simulink model "MultirotorSimPx4v1_8ContMatrix"  (R2018b)
settings: Solver=ode45  StartTime=0.0  StopTime=Simulation.T_END  MaxStep=Simulation.TS_MAX  RelTol=1e-3  EnableMultiTasking=on
PreLoadFcn:
  | % InitializeParameters;
undefined symbols (not defined in the file): Ctrl, Initial, Kpid, Uav, Wind
libraries: QuaternionLibrary x13, simulink x5, simulink_extras x4
(part 2 of 2)

== system MultirotorSimPx4v1_8ContMatrix/Hinf Controller/2D Rotation Matrix ==
  psi : Inport
  Cos : Trigonometry  Operator=cos
  Cos1 : Trigonometry
  Cos2 : Trigonometry
  Cos3 : Trigonometry  Operator=cos
  Gain : Gain  Gain=-1
  Matrix Concatenate : Concatenate  Mode=Multidimensional array  ConcatenateDimension=2
  Mux : Mux  Inputs=2
  Mux1 : Mux  Inputs=2
  R : Outport
  wires:
  Cos3/1 -> Mux1/2
  Cos2/1 -> Mux1/1
  Mux/1 -> Matrix Concatenate/1
  Cos1/1 -> Gain/1
  Cos/1 -> Mux/1
  Gain/1 -> Mux/2
  Mux1/1 -> Matrix Concatenate/2
  Matrix Concatenate/1 -> R/1
  psi/1 -> Cos/1, Cos1/1, Cos2/1, Cos3/1

== system MultirotorSimPx4v1_8ContMatrix/Pos Control/Filtered Derivative ==
  xiDot : Inport  Unit=m/s
  D filter x : TransferFcn  Denominator=[1/(PID_FC*2*pi) 1]  ContinuousStateAttributes='velPID_D_x'
  D filter y : TransferFcn  Denominator=[1/(PID_FC*2*pi) 1]  ContinuousStateAttributes='velPID_D_y'
  D filter z : TransferFcn  Denominator=[1/(PID_FC*2*pi) 1]  ContinuousStateAttributes='velPID_D_z'
  Demux : Demux  Outputs=3
  Mux2 : Mux  Inputs=3
  xiDDotF : Outport  Unit=m/s^2
  wires:
  D filter x/1 -> Mux2/1
  Demux/2 -> D filter y/1
  D filter y/1 -> Mux2/2
  xiDot/1 -> Demux/1
  D filter z/1 -> Mux2/3
  Demux/1 -> D filter x/1
  Demux/3 -> D filter z/1
  Mux2/1 -> xiDDotF/1

== system MultirotorSimPx4v1_8ContMatrix/Pos Control/Filtered Derivative1 ==
  xiDot : Inport  Unit=m/s
  D filter x : TransferFcn  Numerator=[1 0]  Denominator=[1/(PID_FC*2*pi) 1]  ContinuousStateAttributes='velPID_D_x'
  D filter y : TransferFcn  Numerator=[1 0]  Denominator=[1/(PID_FC*2*pi) 1]  ContinuousStateAttributes='velPID_D_y'
  D filter z : TransferFcn  Numerator=[1 0]  Denominator=[1/(PID_FC*2*pi) 1]  ContinuousStateAttributes='velPID_D_z'
  Demux : Demux  Outputs=3
  Mux2 : Mux  Inputs=3
  xiDDotF : Outport  Unit=m/s^2
  wires:
  Mux2/1 -> xiDDotF/1
  Demux/3 -> D filter z/1
  Demux/1 -> D filter x/1
  D filter z/1 -> Mux2/3
  xiDot/1 -> Demux/1
  D filter y/1 -> Mux2/2
  Demux/2 -> D filter y/1
  D filter x/1 -> Mux2/1

== system MultirotorSimPx4v1_8ContMatrix/Pos Control/x vel PID ==
  ref : Inport
  meas : Inport  Port=2
  Add : Sum  Inputs=++-
  D : Gain  Gain=PID_D
  D filter : TransferFcn  Numerator=[1 0]  Denominator=[1/(PID_FC*2*pi) 1]  ContinuousStateAttributes=PID_D_STATENAME
  I : Gain  Gain=PID_I
  Integrator1 : Integrator  UpperSaturationLimit=0.3  LowerSaturationLimit=-0.3  ContinuousStateAttributes=PID_I_STATENAME
  P : Gain  Gain=PID_P
  Sum : Sum  Inputs=|+-
  Out : Outport
  wires:
  Add/1 -> Out/1
  P/1 -> Add/1
  Integrator1/1 -> Add/2
  D filter/1 -> D/1
  Sum/1 -> I/1, P/1
  D/1 -> Add/3
  I/1 -> Integrator1/1
  ref/1 -> Sum/1
  meas/1 -> D filter/1, Sum/2

== system MultirotorSimPx4v1_8ContMatrix/Pos Control/y vel PID ==
  ref : Inport
  meas : Inport  Port=2
  Add : Sum  Inputs=++-
  D : Gain  Gain=PID_D
  D filter : TransferFcn  Numerator=[1 0]  Denominator=[1/(PID_FC*2*pi) 1]  ContinuousStateAttributes=PID_D_STATENAME
  I : Gain  Gain=PID_I
  Integrator1 : Integrator  UpperSaturationLimit=0.3  LowerSaturationLimit=-0.3  ContinuousStateAttributes=PID_I_STATENAME
  P : Gain  Gain=PID_P
  Sum : Sum  Inputs=|+-
  Out : Outport
  wires:
  meas/1 -> Sum/2, D filter/1
  ref/1 -> Sum/1
  I/1 -> Integrator1/1
  D/1 -> Add/3
  Sum/1 -> P/1, I/1
  D filter/1 -> D/1
  Integrator1/1 -> Add/2
  P/1 -> Add/1
  Add/1 -> Out/1

== system MultirotorSimPx4v1_8ContMatrix/Pos Control/z vel PID ==
  ref : Inport
  meas : Inport  Port=2
  Add : Sum  Inputs=++-
  D : Gain  Gain=PID_D
  D filter : TransferFcn  Numerator=[1 0]  Denominator=[1/(PID_FC*2*pi) 1]  ContinuousStateAttributes=PID_D_STATENAME
  I : Gain  Gain=PID_I
  Integrator1 : Integrator  UpperSaturationLimit=0.3  LowerSaturationLimit=-0.3  ContinuousStateAttributes=PID_I_STATENAME
  P : Gain  Gain=PID_P
  Sum : Sum  Inputs=|+-
  Out : Outport
  wires:
  Add/1 -> Out/1
  P/1 -> Add/1
  Integrator1/1 -> Add/2
  D filter/1 -> D/1
  Sum/1 -> I/1, P/1
  D/1 -> Add/3
  I/1 -> Integrator1/1
  ref/1 -> Sum/1
  meas/1 -> D filter/1, Sum/2

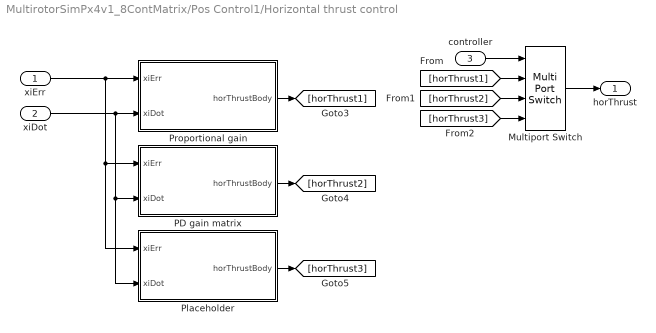
== system MultirotorSimPx4v1_8ContMatrix/Pos Control1/Horizontal thrust control ==
  "xiErr " : Inport
  "xiDot " : Inport  Port=2
  controller : Inport  Port=3
  Multiport Switch : MultiPortSwitch
  PD gain matrix : Subsystem  VariantControl=HorThrustWorldFrame
  Placeholder : Subsystem  VariantControl=HorThrustWorldFrame
  Proportional gain : Subsystem  VariantControl=HorThrustWorldFrame
  " horThrust" : Outport
  wires:
  "xiErr "/1 -> PD gain matrix/1("xiErr "), Placeholder/1("xiErr "), Proportional gain/1("xiErr ")
  "xiDot "/1 -> Proportional gain/2("xiDot "), PD gain matrix/2(xiDot), Placeholder/2(xiDot)
  Multiport Switch/1 -> " horThrust"/1
  controller/1 -> Multiport Switch/1
  Proportional gain/1(" horThrustBody") -> [horThrust1]
  PD gain matrix/1(" horThrustBody") -> [horThrust2]
  Placeholder/1(" horThrustBody") -> [horThrust3]
  [horThrust1] -> Multiport Switch/2
  [horThrust2] -> Multiport Switch/3
  [horThrust3] -> Multiport Switch/4

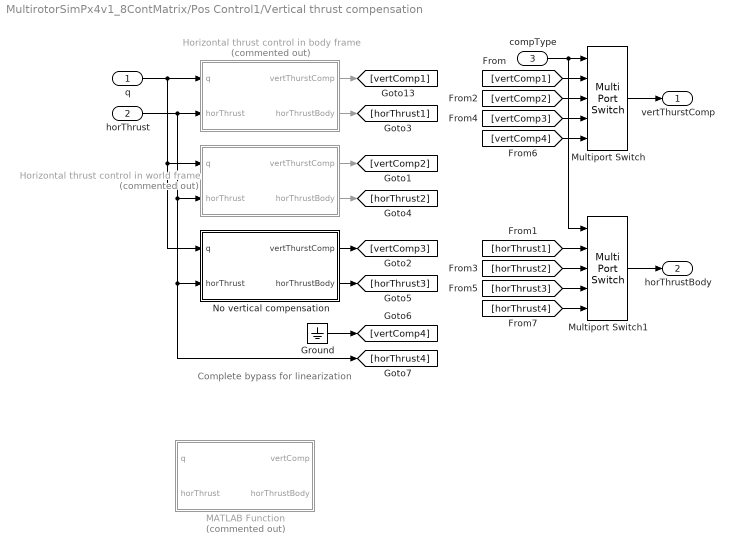
== system MultirotorSimPx4v1_8ContMatrix/Pos Control1/Vertical thrust compensation ==
  note: Complete bypass for linearization
  "q " : Inport
  "horThrust " : Inport  Port=2
  compType : Inport  Port=3
  Ground : Ground
  Horizontal thrust control in body frame : Subsystem  Commented=on  VariantControl=HorThrustBodyFrame
  Horizontal thrust control in world frame : Subsystem  Commented=on  VariantControl=HorThrustWorldFrame
  MATLAB Function : MATLAB Function  Commented=on  TreatAsAtomicUnit=on
  Multiport Switch : MultiPortSwitch  Inputs=4
  Multiport Switch1 : MultiPortSwitch  Inputs=4
  No vertical compensation : Subsystem  VariantControl=HorThrustNoVertComp
  " vertThurstComp" : Outport
  " horThrustBody" : Outport  Port=2
  wires:
  Ground/1 -> [vertComp4]
  [horThrust4] -> Multiport Switch1/5
  [vertComp4] -> Multiport Switch/5
  [horThrust1] -> Multiport Switch1/2
  [horThrust2] -> Multiport Switch1/3
  [horThrust3] -> Multiport Switch1/4
  [vertComp3] -> Multiport Switch/4
  [vertComp2] -> Multiport Switch/3
  [vertComp1] -> Multiport Switch/2
  No vertical compensation/2(" horThrustBody") -> [horThrust3]
  Horizontal thrust control in world frame/2(" horThrustBody") -> [horThrust2]
  Horizontal thrust control in body frame/2(horThrustBody) -> [horThrust1]
  No vertical compensation/1(" vertThurstComp") -> [vertComp3]
  Horizontal thrust control in world frame/1(" vertThurstComp") -> [vertComp2]
  Horizontal thrust control in body frame/1(vertThurstComp) -> [vertComp1]
  compType/1 -> Multiport Switch/1, Multiport Switch1/1
  Multiport Switch1/1 -> " horThrustBody"/1
  Multiport Switch/1 -> " vertThurstComp"/1
  "horThrust "/1 -> Horizontal thrust control in body frame/2(horThrust), Horizontal thrust control in world frame/2("horThrust "), No vertical compensation/2("horThrust "), [horThrust4]
  "q "/1 -> Horizontal thrust control in body frame/1(q), Horizontal thrust control in world frame/1("q "), No vertical compensation/1("q ")

== system MultirotorSimPx4v1_8ContMatrix/Pos Control1/Horizontal thrust control/PD gain matrix ==
  "xiErr " : Inport
  xiDot : Inport  Port=2
  HT_xDotYDot : Gain  Gain=-0.001
  HT_xy : Gain  Gain=0.01
  Selector : Selector  InputPortWidth=3  IndexOptions=Index vector (dialog)  Indices=[1 2]  OutputSizes=1
  Selector1 : Selector  InputPortWidth=3  IndexOptions=Index vector (dialog)  Indices=[1 2]  OutputSizes=1
  Sum : Sum  Inputs=|++
  " horThrustBody" : Outport
  wires:
  Sum/1 -> " horThrustBody"/1
  HT_xDotYDot/1 -> Sum/2
  HT_xy/1 -> Sum/1
  Selector1/1 -> HT_xDotYDot/1
  Selector/1 -> HT_xy/1
  xiDot/1 -> Selector1/1
  "xiErr "/1 -> Selector/1

== system MultirotorSimPx4v1_8ContMatrix/Pos Control1/Horizontal thrust control/Placeholder ==
  "xiErr " : Inport
  xiDot : Inport  Port=2
  C : simulink/Continuous/PID Controller  Controller=PD  Form=Parallel  TimeDomain=Continuous-time  SampleTime=-1  IntegratorMethod=Forward Euler  FilterMethod=Forward Euler  ControllerParametersSource=internal  P=3.97886854580772  I=1  D=0.19015657256146  UseFilter=on  N=18.1835914295571  TunerSelectOption=Transfer Function Based (PID Tuner App)  InitialConditionSource=internal  InitialConditionForIntegrator=0  InitialConditionForFilter=0  DifferentiatorICPrevScaledInput=0  ExternalReset=none  TrackingMode=off  Kt=1  LimitOutput=off  UpperSaturationLimit=inf  LowerSaturationLimit=-inf  LinearizeAsGain=on  AntiWindupMode=none  Kb=1  POutMin=[]  POutMax=[]  IOutMin=[]  IOutMax=[]  DOutMin=[]  DOutMax=[]  NOutMin=[]  NOutMax=[]  SumOutMin=[]  SumOutMax=[]  SaturationOutMin=[]  SaturationOutMax=[]  PParamMin=[]  PParamMax=[]  IParamMin=[]  IParamMax=[]  DParamMin=[]  DParamMax=[]  NParamMin=[]  NParamMax=[]  KbParamMin=[]  KbParamMax=[]  KtParamMin=[]  KtParamMax=[]  KbOutMin=[]  KbOutMax=[]  KtOutMin=[]  KtOutMax=[]  IntegratorOutMin=[]  IntegratorOutMax=[]  FilterOutMin=[]  FilterOutMax=[]  SumI1OutMin=[]  SumI1OutMax=[]  SumI2OutMin=[]  SumI2OutMax=[]  SumI3OutMin=[]  SumI3OutMax=[]  SumI4OutMin=[]  SumI4OutMax=[]  SumDOutMin=[]  SumDOutMax=[]  DifferentiatorOutMin=[]  DifferentiatorOutMax=[]  FilterDiffOutCoefMin=[]  FilterDiffOutCoefMax=[]  ReciprocalOutMin=[]  ReciprocalOutMax=[]  SumDenOutMin=[]  SumDenOutMax=[]  SumNumOutMin=[]  SumNumOutMax=[]  DivideOutMin=[]  DivideOutMax=[]  IntegratorContinuousStateAttributes=''  IntegratorStateMustResolveToSignalObject=off  IntegratorRTWStateStorageClass=Auto  FilterContinuousStateAttributes=''  FilterStateMustResolveToSignalObject=off  FilterRTWStateStorageClass=Auto  ParallelPVariant=InternalParameters  IdealPVariant=Disabled  IVariant=Disabled  DVariant=InternalParameters  IntegratorVariant=Disabled  SatVariant=Disabled  AWVariant=Disabled  PCopyVariant=Disabled  TRVariant=Disabled  FdbkBlocksVariant=Forward  IdealPFdbkVariant=Disabled  SatFdbkVariant=Disabled  DerivativeFilterVariant=ContFilter  NVariant=InternalParameters  NCopyVariant=Disabled  FilterICVariant=InternalICsFilter  IntegratorICVariant=Disabled  ExternalResetVariant=Disabled  TRSumVariant=Passthrough  SumFdbkVariant=Disabled  SumVariant=Sum_PD
  C1 : simulink/Continuous/PID Controller  Controller=PD  Form=Parallel  TimeDomain=Continuous-time  SampleTime=-1  IntegratorMethod=Forward Euler  FilterMethod=Forward Euler  ControllerParametersSource=internal  P=3.97886854580772  I=1  D=0.19015657256146  UseFilter=on  N=18.1835914295571  TunerSelectOption=Transfer Function Based (PID Tuner App)  InitialConditionSource=internal  InitialConditionForIntegrator=0  InitialConditionForFilter=0  DifferentiatorICPrevScaledInput=0  ExternalReset=none  TrackingMode=off  Kt=1  LimitOutput=off  UpperSaturationLimit=inf  LowerSaturationLimit=-inf  LinearizeAsGain=on  AntiWindupMode=none  Kb=1  POutMin=[]  POutMax=[]  IOutMin=[]  IOutMax=[]  DOutMin=[]  DOutMax=[]  NOutMin=[]  NOutMax=[]  SumOutMin=[]  SumOutMax=[]  SaturationOutMin=[]  SaturationOutMax=[]  PParamMin=[]  PParamMax=[]  IParamMin=[]  IParamMax=[]  DParamMin=[]  DParamMax=[]  NParamMin=[]  NParamMax=[]  KbParamMin=[]  KbParamMax=[]  KtParamMin=[]  KtParamMax=[]  KbOutMin=[]  KbOutMax=[]  KtOutMin=[]  KtOutMax=[]  IntegratorOutMin=[]  IntegratorOutMax=[]  FilterOutMin=[]  FilterOutMax=[]  SumI1OutMin=[]  SumI1OutMax=[]  SumI2OutMin=[]  SumI2OutMax=[]  SumI3OutMin=[]  SumI3OutMax=[]  SumI4OutMin=[]  SumI4OutMax=[]  SumDOutMin=[]  SumDOutMax=[]  DifferentiatorOutMin=[]  DifferentiatorOutMax=[]  FilterDiffOutCoefMin=[]  FilterDiffOutCoefMax=[]  ReciprocalOutMin=[]  ReciprocalOutMax=[]  SumDenOutMin=[]  SumDenOutMax=[]  SumNumOutMin=[]  SumNumOutMax=[]  DivideOutMin=[]  DivideOutMax=[]  IntegratorContinuousStateAttributes=''  IntegratorStateMustResolveToSignalObject=off  IntegratorRTWStateStorageClass=Auto  FilterContinuousStateAttributes=''  FilterStateMustResolveToSignalObject=off  FilterRTWStateStorageClass=Auto  ParallelPVariant=InternalParameters  IdealPVariant=Disabled  IVariant=Disabled  DVariant=InternalParameters  IntegratorVariant=Disabled  SatVariant=Disabled  AWVariant=Disabled  PCopyVariant=Disabled  TRVariant=Disabled  FdbkBlocksVariant=Forward  IdealPFdbkVariant=Disabled  SatFdbkVariant=Disabled  DerivativeFilterVariant=ContFilter  NVariant=InternalParameters  NCopyVariant=Disabled  FilterICVariant=InternalICsFilter  IntegratorICVariant=Disabled  ExternalResetVariant=Disabled  TRSumVariant=Passthrough  SumFdbkVariant=Disabled  SumVariant=Sum_PD
  Mux : Mux  Inputs=2
  Selector : Selector  InputPortWidth=3  IndexOptions=Index vector (dialog)  Indices=[1]  OutputSizes=1
  Selector1 : Selector  InputPortWidth=3  IndexOptions=Index vector (dialog)  Indices=[2]  OutputSizes=1
  Terminator1 : Terminator
  " horThrustBody" : Outport
  wires:
  C/1 -> Mux/1  "u"
  C1/1 -> Mux/2  "u"
  Selector/1 -> C/1
  Selector1/1 -> C1/1
  Mux/1 -> " horThrustBody"/1
  xiDot/1 -> Terminator1/1
  "xiErr "/1 -> Selector1/1, Selector/1

== system MultirotorSimPx4v1_8ContMatrix/Pos Control1/Horizontal thrust control/Proportional gain ==
  "xiErr " : Inport
  "xiDot " : Inport  Port=2
  Selector : Selector  InputPortWidth=3  IndexOptions=Index vector (dialog)  Indices=[1 2]  OutputSizes=1
  Terminator : Terminator
  hor_xy : Gain  Gain=Ctrl.HOR_GAIN
  " horThrustBody" : Outport
  wires:
  Selector/1 -> hor_xy/1
  "xiDot "/1 -> Terminator/1
  hor_xy/1 -> " horThrustBody"/1
  "xiErr "/1 -> Selector/1

== system MultirotorSimPx4v1_8ContMatrix/Pos Control1/Vertical thrust compensation/Horizontal thrust control in body frame ==
  q : Inport
  horThrust : Inport  Port=2
  2D Rotation Matrix : Subsystem
  Matrix Multiply : Product  Multiplication=Matrix(*)
  Quaternion to Euler Angles : QuaternionLibrary/Quaternion to Euler Angles
  Selector : Selector  InputPortWidth=3  IndexOptions=Index vector (dialog)  Indices=3  OutputSizes=1
  Subsystem : Subsystem
  vertThurstComp : Outport
  horThrustBody : Outport  Port=2
  wires:
  Matrix Multiply/1 -> horThrustBody/1
  2D Rotation Matrix/1(R) -> Matrix Multiply/1
  Selector/1 -> 2D Rotation Matrix/1(psi)
  Subsystem/1(thrustComp) -> vertThurstComp/1
  Quaternion to Euler Angles/1 -> Selector/1
  q/1 -> Subsystem/1(q), Quaternion to Euler Angles/1
  horThrust/1 -> Subsystem/2(horThrust), Matrix Multiply/2

== system MultirotorSimPx4v1_8ContMatrix/Pos Control1/Vertical thrust compensation/Horizontal thrust control in world frame ==
  "q " : Inport
  "horThrust " : Inport  Port=2
  Demux : Demux  Outputs=3
  Gain : Gain  Commented=through  Gain=-1
  Matrix Multiply1 : Product  Multiplication=Matrix(*)
  Mux : Mux  Inputs=2
  Mux1 : Mux  Inputs=2
  Quaternion to Rotation Matrix : QuaternionLibrary/Quaternion to Rotation Matrix
  Transpose : Math  Operator=transpose  SaturateOnIntegerOverflow=on
  z element : Constant  Value=0
  " vertThurstComp" : Outport
  " horThrustBody" : Outport  Port=2
  wires:
  Transpose/1 -> Matrix Multiply1/1
  Gain/1 -> " vertThurstComp"/1
  Demux/3 -> Gain/1
  Mux1/1 -> " horThrustBody"/1
  Demux/1 -> Mux1/1
  Demux/2 -> Mux1/2
  Matrix Multiply1/1 -> Demux/1  "horThurstBody"
  Quaternion to Rotation Matrix/1 -> Transpose/1
  "q "/1 -> Quaternion to Rotation Matrix/1
  "horThrust "/1 -> Mux/1
  z element/1 -> Mux/2
  Mux/1 -> Matrix Multiply1/2

== system MultirotorSimPx4v1_8ContMatrix/Pos Control1/Vertical thrust compensation/No vertical compensation ==
  "q " : Inport
  "horThrust " : Inport  Port=2
  2D Rotation Matrix : Subsystem
  Ground : Ground
  Matrix Multiply : Product  Multiplication=Matrix(*)
  Quaternion to Euler Angles : QuaternionLibrary/Quaternion to Euler Angles
  Scope : Scope
  Selector : Selector  InputPortWidth=3  IndexOptions=Index vector (dialog)  Indices=3  OutputSizes=1
  " vertThurstComp" : Outport
  " horThrustBody" : Outport  Port=2
  wires:
  "horThrust "/1 -> Matrix Multiply/2
  Quaternion to Euler Angles/1 -> Selector/1
  Selector/1 -> 2D Rotation Matrix/1(psi), Scope/1
  "q "/1 -> Quaternion to Euler Angles/1
  2D Rotation Matrix/1(R) -> Matrix Multiply/1
  Ground/1 -> " vertThurstComp"/1
  Matrix Multiply/1 -> " horThrustBody"/1

== system MultirotorSimPx4v1_8ContMatrix/Pos Control1/Vertical thrust compensation/Horizontal thrust control in body frame/2D Rotation Matrix ==
  psi : Inport
  Cos : Trigonometry  Operator=cos
  Cos1 : Trigonometry
  Cos2 : Trigonometry
  Cos3 : Trigonometry  Operator=cos
  Display : Display
  Gain : Gain  Gain=-1
  Matrix Concatenate : Concatenate  Mode=Multidimensional array  ConcatenateDimension=2
  Mux : Mux  Inputs=2
  Mux1 : Mux  Inputs=2
  R : Outport
  wires:
  psi/1 -> Cos3/1, Cos2/1, Cos1/1, Cos/1
  Matrix Concatenate/1 -> R/1, Display/1
  Mux1/1 -> Matrix Concatenate/2
  Gain/1 -> Mux/2
  Cos/1 -> Mux/1
  Cos1/1 -> Gain/1
  Mux/1 -> Matrix Concatenate/1
  Cos2/1 -> Mux1/1
  Cos3/1 -> Mux1/2

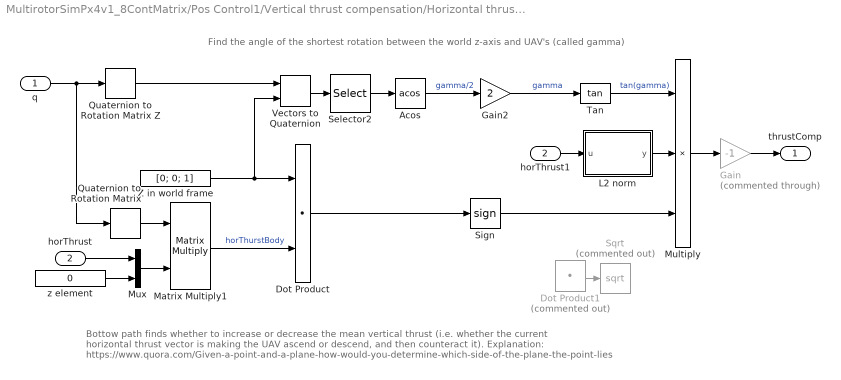
== system MultirotorSimPx4v1_8ContMatrix/Pos Control1/Vertical thrust compensation/Horizontal thrust control in body frame/Subsystem ==
  note: Bottow path finds whether to increase or decrease the mean vertical thrust (i.e. whether the current horizontal thrust vector is
      | making the UAV ascend or descend, and then counteract it).
      | Explanation: https://www.quora.com/Given-a-point-and-a-plane-how-would-you-determine-which-side-of-the-plane-the-point-lies
  note: Find the angle of the shortest rotation between the world z-axis and UAV's (called gamma)
  q : Inport
  horThrust : Inport  Port=2
  Acos : Trigonometry  Operator=acos
  Dot Product : DotProduct  InputSameDT=on  OutDataTypeStr=Inherit: Inherit via internal rule
  Dot Product1 : DotProduct  Commented=on  InputSameDT=on  OutDataTypeStr=Inherit: Inherit via internal rule
  Gain : Gain  Commented=through  Gain=-1
  Gain2 : Gain  Gain=2
  L2 norm : MATLAB Function  TreatAsAtomicUnit=on
  Matrix Multiply1 : Product  Multiplication=Matrix(*)
  Multiply : Product  Inputs=***
  Mux : Mux  Inputs=2
  Quaternion to Rotation Matrix : QuaternionLibrary/Quaternion to Rotation Matrix
  Quaternion to Rotation Matrix Z : QuaternionLibrary/Quaternion to Rotation Matrix Z
  Selector2 : Selector  InputPortWidth=4  IndexOptions=Index vector (dialog)  Indices=1  OutputSizes=1
  Sign : Signum
  Sqrt : Sqrt  Commented=on  SaturateOnIntegerOverflow=on
  Tan : Trigonometry  Operator=tan
  Vectors to Quaternion : QuaternionLibrary/Vectors to Quaternion
  Z in world frame : Constant  Value=[0; 0; 1]
  horThrust1 : InportShadow  Port=2
  z element : Constant  Value=0
  thrustComp : Outport
  wires:
  Dot Product1/1 -> Sqrt/1
  Gain/1 -> thrustComp/1
  L2 norm/1(y) -> Multiply/2
  horThrust1/1 -> L2 norm/1(u)
  Tan/1 -> Multiply/1  "tan(gamma)"
  horThrust/1 -> Mux/1
  Sign/1 -> Multiply/3
  Mux/1 -> Matrix Multiply1/2
  z element/1 -> Mux/2
  Z in world frame/1 -> Dot Product/1, Vectors to Quaternion/2
  q/1 -> Quaternion to Rotation Matrix Z/1, Quaternion to Rotation Matrix/1
  Quaternion to Rotation Matrix/1 -> Matrix Multiply1/1
  Multiply/1 -> Gain/1
  Quaternion to Rotation Matrix Z/1 -> Vectors to Quaternion/1
  Gain2/1 -> Tan/1  "gamma"
  Dot Product/1 -> Sign/1
  Matrix Multiply1/1 -> Dot Product/2  "horThurstBody"
  Acos/1 -> Gain2/1  "gamma/2"
  Vectors to Quaternion/1 -> Selector2/1
  Selector2/1 -> Acos/1

== system MultirotorSimPx4v1_8ContMatrix/Pos Control1/Vertical thrust compensation/No vertical compensation/2D Rotation Matrix ==
  psi : Inport
  Cos : Trigonometry  Operator=cos
  Display : Display
  Gain : Gain  Gain=-1
  Matrix Concatenate : Concatenate  Mode=Multidimensional array  ConcatenateDimension=2
  Mux : Mux  Inputs=2
  Mux1 : Mux  Inputs=2
  Sin : Trigonometry
  R : Outport
  wires:
  psi/1 -> Cos/1, Sin/1
  Matrix Concatenate/1 -> R/1, Display/1
  Mux1/1 -> Matrix Concatenate/2
  Gain/1 -> Mux/2
  Mux/1 -> Matrix Concatenate/1
  Sin/1 -> Gain/1, Mux1/1
  Cos/1 -> Mux/1, Mux1/2

== matlab function MultirotorSimPx4v1_8ContMatrix/Quadrotor Euler Model/Equations of motion ==
  data: VBody input; VBodyDot output; nuBody input; eta input; etaDot input; TBody input size=3; tauBody input size=3; F_D input size=3; M_D input size=3; nuBodyDot output; Uav parameter; xiDDot output; etaDDot output
function [VBodyDot, nuBodyDot, xiDDot, etaDDot] = QuadrotorQuaternionModel(...
    VBody, nuBody, eta, etaDot, TBody, tauBody, F_D, M_D, Uav )
%#codegen

%% Rotation matrices
% Precompute sines and cosines
sPhi   = sin(eta(1));
sTheta = sin(eta(2));
sPsi   = sin(eta(3));
cPhi   = cos(eta(1));
cTheta = cos(eta(2));
cPsi   = cos(eta(3));
tTheta = tan(eta(2));

phiDot   = etaDot(1);
thetaDot = etaDot(2);

% Body frame to inertial frame
R = [cPsi*cTheta, cPsi*sTheta*sPhi-sPsi*cPhi, cPsi*sTheta*cPhi+sPsi*sPhi;
     sPsi*cTheta, sPsi*sTheta*sPhi+cPsi*cPhi, sPsi*sTheta*cPhi-cPsi*sPhi;
     -sTheta,     cTheta*sPhi,                cTheta*cPhi+sPsi*sPhi];

WInvertDot = [...
    0,  phiDot*cPhi*tTheta+thetaDot*sPhi/cTheta^2,    -phiDot*sPhi*cTheta+thetaDot*cPhi/cTheta^2;
    0, -phiDot*sPhi,                                  -phiDot*cPhi;
	0,  phiDot*cPhi/cTheta+phiDot*sPhi*tTheta/cTheta, -phiDot*sPhi/cTheta+thetaDot*cPhi*tTheta/cTheta];

WInvert = [1, sPhi*tTheta,  cPhi*tTheta;
           0, cPhi,        -sPhi;
           0, sPhi/cTheta,  cPhi/cTheta];


%% Moments and Forces
% Body frame accelerations
VBodyDot  = (1/Uav.M) * (R'*Uav.G + TBody - cross(nuBody, Uav.M*VBody) + F_D);
nuBodyDot = Uav.I \ (tauBody - cross(nuBody, Uav.I*nuBody) + M_D);

% Inertial frame accelerations
xiDDot = (1/Uav.M)*(Uav.G + R*TBody + R*F_D);
etaDDot = WInvertDot*nuBody + WInvert*nuBodyDot;

end

== matlab function MultirotorSimPx4v1_8ContMatrix/Subsystem1/MATLAB Function ==
  data: q input; rates_sp output; qd input; thrust_sp input; yaw_sp_move_rate input; attitude_gain input; auto_rate_max input
function rates_sp  = control_attitude( q, qd, thrust_sp, ...
    yaw_sp_move_rate, attitude_gain, auto_rate_max )

%thrust_sp = -thrust_sp;

roll_pitch_gain = ( attitude_gain(1) + attitude_gain(2) ) / 2;
yaw_w = constrain( attitude_gain(3) / roll_pitch_gain, 0, 1 );
attitude_gain(3) = roll_pitch_gain;

q  = q  ./ norm(q);
qd = qd ./ norm(qd);

e_z   = QuatToDcmZ( q );
e_z_d = QuatToDcmZ( qd );
qd_red = VecsToQuat( e_z, e_z_d );

qd_red = QuatMult( qd_red, q );

q_mix = QuatMult( InvertQuat(qd_red), qd );
q_mix = q_mix .* SignNoZero( q_mix(1) );

q_mix(1) = constrain( q_mix(1), -1, 1 );
q_mix(4) = constrain( q_mix(4), -1, 1 );
qd = QuatMult( qd_red, ...
    [ cos( yaw_w * acos(q_mix(1)) );
    0;
    0;
    sin( yaw_w * asin(q_mix(4)) ) ] );

qe = QuatMult( InvertQuat(q), qd );

eq = 2 .* SignNoZero(qe(1)) .* qe(2:4);

rates_sp = eq .* attitude_gain;

rates_sp = rates_sp + QuatToDcmZ( InvertQuat(q) ) .* yaw_sp_move_rate;

rates_sp = constrain( rates_sp, -auto_rate_max, auto_rate_max);
end

function y = constrain( x, x_min, x_max )
    y = max( min(x, x_max), x_min );
end

function dcmZ = QuatToDcmZ( quat )
    a = quat(1);
    b = quat(2);
    c = quat(3);
    d = quat(4);
    dcmZ = [ 2 * (a * c + b * d);
        2 * (c * d - a * b);
        a * a - b * b - c * c + d * d ];
end

function quat = VecsToQuat( src, dst )
    cr = cross(src, dst);
    dt = dot(src, dst);
    quat = zeros(4,1);
    locEps = 1e-5; % Don't use eps as it's a reserved variable in MATLAB
    if (norm(cr) < locEps && dt < 0)
        % Handle corner cases with 180 degree rotations
        % If the two vectors are parallel, cross product is zero
        % If they point opposite, the dot product is negative
        cr = abs(src);
        if (cr(1) < cr(2))
            if (cr(1) < cr(3))
                cr = [1; 0; 0];
            else
                cr = [0; 0; 1];
            end
        else
            if (cr(2) < cr(3))
                cr = [0; 1; 0];
            else
                cr = [0; 0; 1];
            end
        end
        quat(1) = 0;
        cr = cross(src, cr);
    else
        % Normal case, do half-way quaternion solution
        quat(1) = dt + sqrt( norm(src)^2 * norm(dst)^2 );
    end
    quat(2) = cr(1);
    quat(3) = cr(2);
    quat(4) = cr(3);
    quat = MulticopterAttitudeControl.normalize( quat );
end

function quatInv = InvertQuat( quat )
    normSq = dot( quat, quat );
    quatInv = ( quat .* [1;-1;-1;-1] ./ normSq );
end

function quatOut = QuatMult( q1, q2 )
    quatOut = [ q1(1) * q2(1) - q1(2) * q2(2) - q1(3) * q2(3) - q1(4) * q2(4) ;
        q1(1) * q2(2) + q1(2) * q2(1) + q1(3) * q2(4) - q1(4) * q2(3) ;
        q1(1) * q2(3) - q1(2) * q2(4) + q1(3) * q2(1) + q1(4) * q2(2) ;
        q1(1) * q2(4) + q1(2) * q2(3) - q1(3) * q2(2) + q1(4) * q2(1) ];
end

function out = SignNoZero( in )
    out = ( 0 <= in ) - ( in < 0 );
end

== matlab function MultirotorSimPx4v1_8ContMatrix/Subsystem1/MATLAB Function1 ==
  data: rate_p input; rate_i input; rate_d input; rates input; att_control output; rates_prev_filtered output; rates_sp input size=3; thrust_sp input; rates_filtered input size=3; rates_prev_filtered input size=3; rates_int output; rates_int input size=3
function [att_control, rates_prev_filtered, rates_int] = control_attitude_rates( rate_p, rate_i, rate_d, ...
    rates, rates_sp, thrust_sp, rates_filtered, rates_prev_filtered, rates_int )

    % values
    rate_int_lim = [ 0.3; 0.3; 0.3 ];
    tpa_breakpoint_p = 1;
    tpa_breakpoint_i = 1;
    tpa_breakpoint_d = 1;
    tpa_rate_p = 0;
    tpa_rate_i = 0;
    tpa_rate_d = 0;
    dt = 1/250;
    rate_ff = zeros(3,1);
    
    rates_p_scaled = rate_p .* pid_attenuations( tpa_breakpoint_p, tpa_rate_p, thrust_sp );
    rates_i_scaled = rate_i .* pid_attenuations( tpa_breakpoint_i, tpa_rate_i, thrust_sp );
    rates_d_scaled = rate_d .* pid_attenuations( tpa_breakpoint_d, tpa_rate_d, thrust_sp );

    rates_err = rates_sp - rates;

    %rates_filtered = LowPassFilter2pVector3Apply( obj, rates );

    att_control = rates_p_scaled .* rates_err + ...
        rates_int - ...
        rates_d_scaled .* (rates_filtered - rates_prev_filtered) / dt + ...
        rate_ff .* rates_sp;

    rates_prev_filtered = rates_filtered;

    rate_i_tmp = rates_int + rates_i_scaled .* rates_err .* dt;
    
    toKeep = isfinite(rate_i_tmp) & (rate_i_tmp > -rate_int_lim) & ...
                (rate_i_tmp < rate_int_lim);
    %rates_int = zeros(3,1);
    rates_int(toKeep) = rate_i_tmp(toKeep);
    
    rates_int = constrain( rates_int, -rate_int_lim, rate_int_lim );
end

function pidAttenuationPerAxis = pid_attenuations( tpa_breakpoint, tpa_rate, thrust_sp )
    TPA_RATE_LOWER_LIMIT = 0.05;
    tpa = 1.0 - tpa_rate * (abs(thrust_sp) - tpa_breakpoint) / (1.0 - tpa_breakpoint);
    tpa = max([TPA_RATE_LOWER_LIMIT, min([1.0, tpa])]);
    pidAttenuationPerAxis = [ tpa; tpa; 1.0 ];
end

function y = constrain( x, x_min, x_max )
    y = max( min(x, x_max), x_min );
end

== matlab function MultirotorSimPx4v1_8ContMatrix/Applied wind speed/Relative velocity ==
  data: nuBody input; Uav parameter; VMotorRelBody output
function VMotorRelBody = relativeMotorVelocity( nuBody , Uav )
%#codegen
    VMotorRelBody = cross( nuBody, Uav.L_VEC );
end

== matlab function MultirotorSimPx4v1_8ContMatrix/Applied wind speed/Compute V_app2 ==
  data: Q input; UBody output; U input size=3
function UBody = computeUBody(Q, U)
%#codegen

% Rotation matrix from Wind frame to Inertial frame
% Wind frame SEU, inertial frame NED
R_U = [1,  0, 0;
       0, -1, 0;
       0,  0, 1];
   
UBody = Q' * R_U * U;

== matlab function MultirotorSimPx4v1_8ContMatrix/Attitude Controller/Attitude loop (nonlinear P control) ==
  data: q input; rates_sp output; qd input; thrust_sp input; yaw_sp_move_rate input; attitude_gain input; auto_rate_max input
function rates_sp  = control_attitude( q, qd, thrust_sp, ...
    yaw_sp_move_rate, attitude_gain, auto_rate_max )
    %thrust_sp = -thrust_sp;

    roll_pitch_gain = ( attitude_gain(1) + attitude_gain(2) ) / 2;
    yaw_w = constrain( attitude_gain(3) / roll_pitch_gain, 0, 1 );
    attitude_gain(3) = roll_pitch_gain;

    q  = q  ./ norm(q);
    qd = qd ./ norm(qd);

    e_z   = QuatToDcmZ( q );
    e_z_d = QuatToDcmZ( qd );
    qd_red = VecsToQuat( e_z, e_z_d );

    qd_red = QuatMult( qd_red, q );

    q_mix = QuatMult( InvertQuat(qd_red), qd );
    q_mix = q_mix .* SignNoZero( q_mix(1) );

    q_mix(1) = constrain( q_mix(1), -1, 1 );
    q_mix(4) = constrain( q_mix(4), -1, 1 );
    qd = QuatMult( qd_red, ...
        [ cos( yaw_w * acos(q_mix(1)) );
        0;
        0;
        sin( yaw_w * asin(q_mix(4)) ) ] );

    qe = QuatMult( InvertQuat(q), qd );

    eq = 2 .* SignNoZero(qe(1)) .* qe(2:4);

    rates_sp = eq .* attitude_gain;

    rates_sp = rates_sp + QuatToDcmZ( InvertQuat(q) ) .* yaw_sp_move_rate;

    rates_sp = constrain( rates_sp, -auto_rate_max, auto_rate_max);
end

function y = constrain( x, x_min, x_max )
    y = max( min(x, x_max), x_min );
end

function dcmZ = QuatToDcmZ( quat )
    a = quat(1);
    b = quat(2);
    c = quat(3);
    d = quat(4);
    dcmZ = [ 2 * (a * c + b * d);
        2 * (c * d - a * b);
        a * a - b * b - c * c + d * d ];
end

function quat = VecsToQuat( src, dst )
    cr = cross(src, dst);
    dt = dot(src, dst);
    quat = zeros(4,1);
    locEps = 1e-5; % Don't use eps as it's a reserved variable in MATLAB
    if (norm(cr) < locEps && dt < 0)
        % Handle corner cases with 180 degree rotations
        % If the two vectors are parallel, cross product is zero
        % If they point opposite, the dot product is negative
        cr = abs(src);
        if (cr(1) < cr(2))
            if (cr(1) < cr(3))
                cr = [1; 0; 0];
            else
                cr = [0; 0; 1];
            end
        else
            if (cr(2) < cr(3))
                cr = [0; 1; 0];
            else
                cr = [0; 0; 1];
            end
        end
        quat(1) = 0;
        cr = cross(src, cr);
    else
        % Normal case, do half-way quaternion solution
        quat(1) = dt + sqrt( norm(src)^2 * norm(dst)^2 );
    end
    quat(2) = cr(1);
    quat(3) = cr(2);
    quat(4) = cr(3);
    quat = MulticopterAttitudeControl.normalize( quat );
end

function quatInv = InvertQuat( quat )
    normSq = dot( quat, quat );
    quatInv = ( quat .* [1;-1;-1;-1] ./ normSq );
end

function quatOut = QuatMult( q1, q2 )
    quatOut = [ q1(1) * q2(1) - q1(2) * q2(2) - q1(3) * q2(3) - q1(4) * q2(4) ;
        q1(1) * q2(2) + q1(2) * q2(1) + q1(3) * q2(4) - q1(4) * q2(3) ;
        q1(1) * q2(3) - q1(2) * q2(4) + q1(3) * q2(1) + q1(4) * q2(2) ;
        q1(1) * q2(4) + q1(2) * q2(3) - q1(3) * q2(2) + q1(4) * q2(1) ];
end

function out = SignNoZero( in )
    out = ( 0 <= in ) - ( in < 0 );
end

== matlab function MultirotorSimPx4v1_8ContMatrix/Pos Control/MATLAB Function ==
  data: thr_sp input size=3; q_sp output; yaw_sp input; thrust_sp output
function [q_sp, thrust_sp] = thrustToAttitude( thr_sp, yaw_sp )

    yaw_body = yaw_sp;
    body_z = -thr_sp./norm(thr_sp);
    
    y_C = [ -sin(yaw_body); cos(yaw_body); 0 ];
    
    body_x = zeros(3,1);
    if body_z(3) > 0.000001
        body_x = cross( y_C, body_z );
        if ( body_z(3) < 0 )
            body_x = -body_x;
        end
        
        body_x = body_x ./ norm(body_x);
    else
        body_x(3) = 1;
    end
    
    body_y = cross( body_z, body_x );
    
    R_sp = [ body_x, body_y, body_z ];
    
    q_sp = from_dcm( R_sp );
    
    thrust_sp = -norm( thr_sp );
    
end

function data  = from_dcm( dcm )
% FROM_DCM Convert DCM to quaternion
% From https://github.com/PX4/Firmware/blob/master/src/lib/mathlib/math/Quaternion.hpp
    data = zeros(4,1);
    tr = dcm(1,1) + dcm(2,2) + dcm(3,3);
    if (tr > 0.0)
        s = sqrt(tr + 1.0);
        data(1) = s * 0.5;
        s = 0.5 / s;
        data(2) = (dcm(3,2) - dcm(2,3) ) * s;
        data(3) = (dcm(1,3) - dcm(3,1) ) * s;
        data(4) = (dcm(2,1) - dcm(1,2) ) * s;
    else
        % Find maximum diagonal element in dcm
        % store index in dcm_i
        dcm_i = 1;
        for i = 2:3 % (int i = 1; i < 3; i++)
            if ( dcm(i,i) > dcm(dcm_i,dcm_i) )
                dcm_i = i;
            end
        end
        dcm_j = rem( ( (dcm_i-1) + 1), 3) + 1;
        dcm_k = rem( ( (dcm_i-1) + 2), 3) + 1;
        s = sqrt( (dcm(dcm_i, dcm_i) - dcm(dcm_j, dcm_j) - ...
            dcm(dcm_k,dcm_k)) + 1.0 );
        data(dcm_i + 1) = s * 0.5;
        s = 0.5 / s;
        data(dcm_j + 1) = ( dcm(dcm_i,dcm_j) + dcm(dcm_j,dcm_i) ) * s;
        data(dcm_k + 1) = ( dcm(dcm_k,dcm_i) + dcm(dcm_i,dcm_k) ) * s;
        data(1) = ( dcm(dcm_k,dcm_j) - dcm(dcm_j,dcm_k) ) * s;
    end
end

== matlab function MultirotorSimPx4v1_8ContMatrix/Compute Sph ==
  data: in input; beta output; alpha output; R output
function [beta, alpha, R] = computeSph(in)
%#codegen

% Convert from polar to spherical coordinates
[ beta, alpha, R ] = cart2sph( in(1), in(2), in(3) );

== matlab function MultirotorSimPx4v1_8ContMatrix/Subsystem2/MATLAB Function ==
  data: q input; rates_sp output; qd input; thrust_sp input; yaw_sp_move_rate input; attitude_gain input; auto_rate_max input
function rates_sp  = control_attitude( q, qd, thrust_sp, ...
    yaw_sp_move_rate, attitude_gain, auto_rate_max )

%thrust_sp = -thrust_sp;

roll_pitch_gain = ( attitude_gain(1) + attitude_gain(2) ) / 2;
yaw_w = constrain( attitude_gain(3) / roll_pitch_gain, 0, 1 );
attitude_gain(3) = roll_pitch_gain;

q  = q  ./ norm(q);
qd = qd ./ norm(qd);

e_z   = QuatToDcmZ( q );
e_z_d = QuatToDcmZ( qd );
qd_red = VecsToQuat( e_z, e_z_d );

qd_red = QuatMult( qd_red, q );

q_mix = QuatMult( InvertQuat(qd_red), qd );
q_mix = q_mix .* SignNoZero( q_mix(1) );

q_mix(1) = constrain( q_mix(1), -1, 1 );
q_mix(4) = constrain( q_mix(4), -1, 1 );
qd = QuatMult( qd_red, ...
    [ cos( yaw_w * acos(q_mix(1)) );
    0;
    0;
    sin( yaw_w * asin(q_mix(4)) ) ] );

qe = QuatMult( InvertQuat(q), qd );

eq = 2 .* SignNoZero(qe(1)) .* qe(2:4);

rates_sp = eq .* attitude_gain;

rates_sp = rates_sp + QuatToDcmZ( InvertQuat(q) ) .* yaw_sp_move_rate;

rates_sp = constrain( rates_sp, -auto_rate_max, auto_rate_max);
end

function y = constrain( x, x_min, x_max )
    y = max( min(x, x_max), x_min );
end

function dcmZ = QuatToDcmZ( quat )
    a = quat(1);
    b = quat(2);
    c = quat(3);
    d = quat(4);
    dcmZ = [ 2 * (a * c + b * d);
        2 * (c * d - a * b);
        a * a - b * b - c * c + d * d ];
end

function quat = VecsToQuat( src, dst )
    cr = cross(src, dst);
    dt = dot(src, dst);
    quat = zeros(4,1);
    locEps = 1e-5; % Don't use eps as it's a reserved variable in MATLAB
    if (norm(cr) < locEps && dt < 0)
        % Handle corner cases with 180 degree rotations
        % If the two vectors are parallel, cross product is zero
        % If they point opposite, the dot product is negative
        cr = abs(src);
        if (cr(1) < cr(2))
            if (cr(1) < cr(3))
                cr = [1; 0; 0];
            else
                cr = [0; 0; 1];
            end
        else
            if (cr(2) < cr(3))
                cr = [0; 1; 0];
            else
                cr = [0; 0; 1];
            end
        end
        quat(1) = 0;
        cr = cross(src, cr);
    else
        % Normal case, do half-way quaternion solution
        quat(1) = dt + sqrt( norm(src)^2 * norm(dst)^2 );
    end
    quat(2) = cr(1);
    quat(3) = cr(2);
    quat(4) = cr(3);
    quat = MulticopterAttitudeControl.normalize( quat );
end

function quatInv = InvertQuat( quat )
    normSq = dot( quat, quat );
    quatInv = ( quat .* [1;-1;-1;-1] ./ normSq );
end

function quatOut = QuatMult( q1, q2 )
    quatOut = [ q1(1) * q2(1) - q1(2) * q2(2) - q1(3) * q2(3) - q1(4) * q2(4) ;
        q1(1) * q2(2) + q1(2) * q2(1) + q1(3) * q2(4) - q1(4) * q2(3) ;
        q1(1) * q2(3) - q1(2) * q2(4) + q1(3) * q2(1) + q1(4) * q2(2) ;
        q1(1) * q2(4) + q1(2) * q2(3) - q1(3) * q2(2) + q1(4) * q2(1) ];
end

function out = SignNoZero( in )
    out = ( 0 <= in ) - ( in < 0 );
end

== matlab function MultirotorSimPx4v1_8ContMatrix/Subsystem2/MATLAB Function1 ==
  data: rate_p input; rate_i input; rate_d input; rates input; att_control output; rates_prev_filtered output; rates_sp input size=3; thrust_sp input; rates_filtered input size=3; rates_prev_filtered input size=3; rates_int output; rates_int input size=3
function [att_control, rates_prev_filtered, rates_int] = control_attitude_rates( rate_p, rate_i, rate_d, ...
    rates, rates_sp, thrust_sp, rates_filtered, rates_prev_filtered, rates_int )

    % values
    rate_int_lim = [ 0.3; 0.3; 0.3 ];
    tpa_breakpoint_p = 1;
    tpa_breakpoint_i = 1;
    tpa_breakpoint_d = 1;
    tpa_rate_p = 0;
    tpa_rate_i = 0;
    tpa_rate_d = 0;
    dt = 1/250;
    rate_ff = zeros(3,1);
    
    rates_p_scaled = rate_p .* pid_attenuations( tpa_breakpoint_p, tpa_rate_p, thrust_sp );
    rates_i_scaled = rate_i .* pid_attenuations( tpa_breakpoint_i, tpa_rate_i, thrust_sp );
    rates_d_scaled = rate_d .* pid_attenuations( tpa_breakpoint_d, tpa_rate_d, thrust_sp );

    rates_err = rates_sp - rates;

    %rates_filtered = LowPassFilter2pVector3Apply( obj, rates );

    att_control = rates_p_scaled .* rates_err + ...
        rates_int - ...
        rates_d_scaled .* (rates_filtered - rates_prev_filtered) / dt + ...
        rate_ff .* rates_sp;

    rates_prev_filtered = rates_filtered;

    rate_i_tmp = rates_int + rates_i_scaled .* rates_err .* dt;
    
    toKeep = isfinite(rate_i_tmp) & (rate_i_tmp > -rate_int_lim) & ...
                (rate_i_tmp < rate_int_lim);
    %rates_int = zeros(3,1);
    rates_int(toKeep) = rate_i_tmp(toKeep);
    
    rates_int = constrain( rates_int, -rate_int_lim, rate_int_lim );
end

function pidAttenuationPerAxis = pid_attenuations( tpa_breakpoint, tpa_rate, thrust_sp )
    TPA_RATE_LOWER_LIMIT = 0.05;
    tpa = 1.0 - tpa_rate * (abs(thrust_sp) - tpa_breakpoint) / (1.0 - tpa_breakpoint);
    tpa = max([TPA_RATE_LOWER_LIMIT, min([1.0, tpa])]);
    pidAttenuationPerAxis = [ tpa; tpa; 1.0 ];
end

function y = constrain( x, x_min, x_max )
    y = max( min(x, x_max), x_min );
end

== matlab function MultirotorSimPx4v1_8ContMatrix/Subsystem2/MATLAB Function2 ==
  data: sample input; output output; delay_element_1 input size=3; delay_element_2 input size=3; delay_element_1 output; delay_element_2 output
function [output, delay_element_1, delay_element_2]  = LowPassFilter2pVector3( sample, delay_element_1, delay_element_2 )
    sample_freq = 250;
    cutoff_freq = 30;
    [a1, a2, b0, b1, b2] = init(sample_freq, cutoff_freq);
    delay_element_0 = sample - delay_element_1.*a1 - delay_element_2.*a2;
    output = delay_element_0.*b0 + delay_element_1.*b1 + delay_element_2.*b2;
    delay_element_2 = delay_element_1;
    delay_element_1 = delay_element_0;
end

function [a1, a2, b0, b1, b2] = init(sample_freq, cutoff_freq)
    fr = sample_freq / cutoff_freq;
    ohm = tan( pi / fr);
    c = 1.0 + 2.0 * cos( pi / 4.0) * ohm + ohm * ohm;

    b0 = ohm * ohm / c;
    b1 = 2.0 * b0;
    b2 = b0;

    a1 = 2.0 * (ohm * ohm - 1.0) / c;
    a2 = (1.0 - 2.0 * cos(pi / 4.0) * ohm + ohm * ohm) / c;
end

== matlab function MultirotorSimPx4v1_8ContMatrix/Quadrotor Euler Model/Compute etaDot ==
  data: nuBody input; eta input; etaDot output
function etaDot = computeEtaDot(nuBody, eta)
%#codegen

sPhi = sin(eta(1));
cPhi = cos(eta(1));
cTheta = cos(eta(2));
tTheta = tan(eta(2));
      
WInverse = [1, sPhi*tTheta,  cPhi*tTheta;
            0, cPhi,        -sPhi;
            0, sPhi/cTheta,  cPhi/cTheta];

etaDot = WInverse*nuBody;

== matlab function MultirotorSimPx4v1_8ContMatrix/Quadrotor Euler Model/compute VBody ==
  data: eta input; VBody output; xiDot input
function VBody = computeVBody(eta, xiDot)
%#codegen

sphi = sin(eta(1));
sTheta = sin(eta(2));
sPsi = sin(eta(3));
cPhi = cos(eta(1));
cTheta = cos(eta(2));
cPsi = cos(eta(3));

R = [ cPsi*cTheta, cPsi*sTheta*sphi-sPsi*cPhi, cPsi*sTheta*cPhi+sPsi*sphi;
	  sPsi*cTheta, sPsi*sTheta*sphi+cPsi*cPhi, sPsi*sTheta*cPhi-cPsi*sphi;
     -sTheta,      cTheta*sphi,                cTheta*cPhi+sPsi*sphi];

VBody = R'*xiDot;

== matlab function MultirotorSimPx4v1_8ContMatrix/L2 norm ==
  data: u input; y output
function y = l2norm( u )
    y = sqrt( dot(u, u) );
end

== matlab function MultirotorSimPx4v1_8ContMatrix/Pos Control1/MATLAB Function ==
  data: thr_sp input size=3; q_sp output; yaw_sp input; thrust_sp output
function [q_sp, thrust_sp] = thrustToAttitude( thr_sp, yaw_sp )

    yaw_body = yaw_sp;
    body_z = -thr_sp./norm(thr_sp);
    
    y_C = [ -sin(yaw_body); cos(yaw_body); 0 ];
    
    body_x = zeros(3,1);
    if body_z(3) > 0.000001
        body_x = cross( y_C, body_z );
        if ( body_z(3) < 0 )
            body_x = -body_x;
        end
        
        body_x = body_x ./ norm(body_x);
    else
        body_x(3) = 1;
    end
    
    body_y = cross( body_z, body_x );
    
    R_sp = [ body_x, body_y, body_z ];
    
    q_sp = from_dcm( R_sp );
    
    thrust_sp = -norm( thr_sp );
    
end

function data  = from_dcm( dcm )
% FROM_DCM Convert DCM to quaternion
% From https://github.com/PX4/Firmware/blob/master/src/lib/mathlib/math/Quaternion.hpp
    data = zeros(4,1);
    tr = dcm(1,1) + dcm(2,2) + dcm(3,3);
    if (tr > 0.0)
        s = sqrt(tr + 1.0);
        data(1) = s * 0.5;
        s = 0.5 / s;
        data(2) = (dcm(3,2) - dcm(2,3) ) * s;
        data(3) = (dcm(1,3) - dcm(3,1) ) * s;
        data(4) = (dcm(2,1) - dcm(1,2) ) * s;
    else
        % Find maximum diagonal element in dcm
        % store index in dcm_i
        dcm_i = 1;
        for i = 2:3 % (int i = 1; i < 3; i++)
            if ( dcm(i,i) > dcm(dcm_i,dcm_i) )
                dcm_i = i;
            end
        end
        dcm_j = rem( ( (dcm_i-1) + 1), 3) + 1;
        dcm_k = rem( ( (dcm_i-1) + 2), 3) + 1;
        s = sqrt( (dcm(dcm_i, dcm_i) - dcm(dcm_j, dcm_j) - ...
            dcm(dcm_k,dcm_k)) + 1.0 );
        data(dcm_i + 1) = s * 0.5;
        s = 0.5 / s;
        data(dcm_j + 1) = ( dcm(dcm_i,dcm_j) + dcm(dcm_j,dcm_i) ) * s;
        data(dcm_k + 1) = ( dcm(dcm_k,dcm_i) + dcm(dcm_i,dcm_k) ) * s;
        data(1) = ( dcm(dcm_k,dcm_j) - dcm(dcm_j,dcm_k) ) * s;
    end
end

== matlab function MultirotorSimPx4v1_8ContMatrix/Pos Control1/Vertical thrust compensation/Horizontal thrust control in body frame/Subsystem/L2 norm ==
  data: u input; y output
function y = l2norm( u )
    y = sqrt( dot(u, u) );
end

== matlab function MultirotorSimPx4v1_8ContMatrix/Pos Control1/Vertical thrust compensation/MATLAB Function ==
  data: vertComp output; q input; horThrustBody output; horThrust input
function [vertComp, horThrustBody] = rotate(q, horThrust)
    eul = QuatToEuler( q );
    psi = eul(3);
    rotMat = [ cos(psi), -sin(psi); sin(psi), cos(psi) ];
    horThrustBody = rotMat * horThrust;
    vertComp = 0;
end

function [ eul ] = QuatToEuler( quat )
%QUATTOEULER Convert quaternion to euler angles (roll, pitch, yaw)
%   Based on PX4 Firmware code
%   Written by: J.X.J. Bannwarth, 07/08/2017

    eul = [ atan2(2.0 .* (quat(1) .* quat(2) + quat(3) .* quat(4)), ...
                1.0 - 2.0 .* (quat(2) .* quat(2) + quat(3) .* quat(3)));
            asin(2.0 .* (quat(1) .* quat(3) - quat(4) .* quat(2)));
            atan2(2.0 .* (quat(1) .* quat(4) + quat(2) .* quat(3)), ...
                1.0 - 2.0 .* (quat(3) .* quat(3) + quat(4) .* quat(4))) ];    
end
